simulink model "lab4_feedforward"  (R2023b)
settings: Solver=ode45  StartTime=0.0  StopTime=150  RelTol=1e-3
settings Model: Creator=Daniela  LastModifiedBy=Daniela

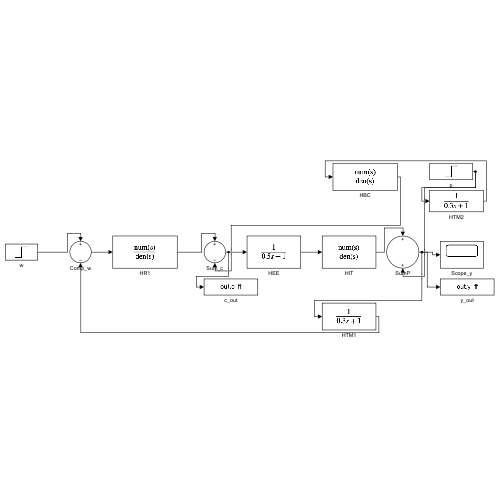
[thumbnail: Simulink's stored preview of the top-level diagram]
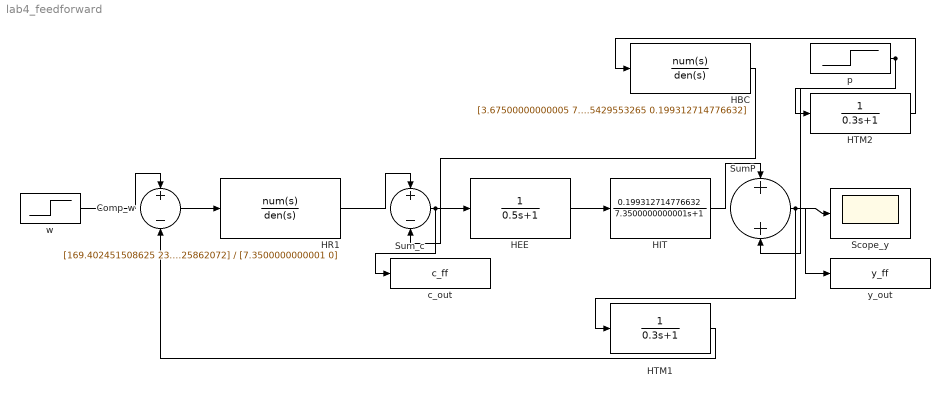
== system lab4_feedforward ==
  Comp_w : Sum  Inputs=+-
  HBC : TransferFcn  Numerator=[3.67500000000005 7.8500000000001 1]  Denominator=[0.00199312714776632 0.0398625429553265 0.199312714776632]
  HEE : TransferFcn  Numerator=1  Denominator=[0.5 1]
  HIT : TransferFcn  Numerator=0.199312714776632  Denominator=[7.3500000000001 1]
  HR1 : TransferFcn  Numerator=[169.402451508625 23.0479525862072]  Denominator=[7.3500000000001 0]
  HTM1 : TransferFcn  Numerator=1  Denominator=[0.3 1]
  HTM2 : TransferFcn  Numerator=1  Denominator=[0.3 1]
  Scope_y : Scope
  SumP : Sum
  Sum_c : Sum  Inputs=+-
  c_out : ToWorkspace  VariableName=c_ff  SampleTime=-1
  p : Step  Time=50  SampleTime=0
  w : Step  Time=0  SampleTime=0
  y_out : ToWorkspace  VariableName=y_ff  SampleTime=-1
  wires:
  w/1 -> Comp_w/1
  Comp_w/1 -> HR1/1
  HR1/1 -> Sum_c/1
  Sum_c/1 -> HEE/1, c_out/1
  HEE/1 -> HIT/1
  HIT/1 -> SumP/1
  p/1 -> SumP/2, HTM2/1
  HTM2/1 -> HBC/1
  HBC/1 -> Sum_c/2
  SumP/1 -> Scope_y/1, y_out/1, HTM1/1
  HTM1/1 -> Comp_w/2
